simulink model "sl_fforward"  (Simulink 7.6)
settings: Solver=ode45  StartTime=0.0  StopTime=10.0  RelTol=1e-3
undefined symbols (not defined in the file or in its folder): p560
libraries: roblocks x4
settings Model: Creator=corkep  LastModifiedBy=n6334687

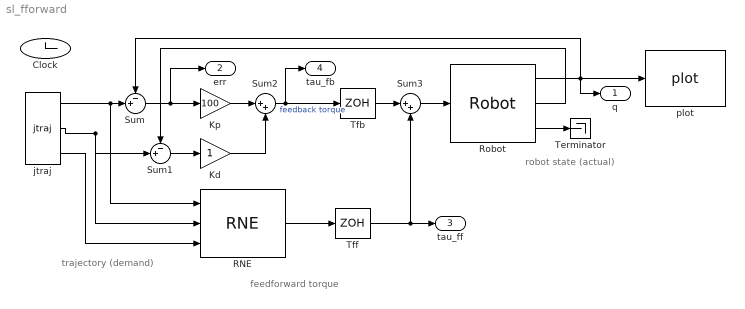
== system sl_fforward ==
  note: trajectory
      | (demand)
  note: robot state
      | (actual)
  note: feedforward torque
  Clock : Clock
      settings: Decimation=10
  Kd : Gain  SaturateOnIntegerOverflow=on  OutDataTypeStr=Inherit: Same as input  ParamDataTypeStr=Inherit: Same as input
  Kp : Gain  Gain=100  SaturateOnIntegerOverflow=on  OutDataTypeStr=Inherit: Same as input  ParamDataTypeStr=Inherit: Same as input
  RNE : roblocks/Dynamics/RNE  SystemSampleTime=-1  robot=p560.nofriction()  grav=[0 0 9.81]
  Robot : roblocks/Dynamics/Robot  SystemSampleTime=-1  robot=p560  q0=[0 0 0 0 0 0]
  Sum : Sum  Inputs=-+|  SaturateOnIntegerOverflow=on  InputSameDT=on  OutDataTypeStr=Inherit: Same as first input
  Sum1 : Sum  Inputs=-+|  SaturateOnIntegerOverflow=on  InputSameDT=on  OutDataTypeStr=Inherit: Same as first input
  Sum2 : Sum  Inputs=|++  SaturateOnIntegerOverflow=on  InputSameDT=on  OutDataTypeStr=Inherit: Same as first input
  Sum3 : Sum  Inputs=|++  SaturateOnIntegerOverflow=on  InputSameDT=on  OutDataTypeStr=Inherit: Same as first input
  Terminator : Terminator
  Tfb : ZeroOrderHold  SampleTime=0.01
  Tff : ZeroOrderHold  SampleTime=0.01
  jtraj : roblocks/Trajectory/jtraj  SystemSampleTime=-1  q0=[0 0 0 0 0 0]  qf=[pi/4 pi/2 -pi/2 0 0 0]  tmax=10
  plot : roblocks/Robot Graphics/plot  SystemSampleTime=-1  robot=p560
  q : Outport
  err : Outport  Port=2
  tau_ff : Outport  Port=3
  tau_fb : Outport  Port=4
  wires:
  Kd/1 -> Sum2/2
  Sum/1 -> Kp/1, err/1
  Kp/1 -> Sum2/1
  Sum1/1 -> Kd/1
  Sum2/1 -> Tfb/1, tau_fb/1  "feedback torque"
  Sum3/1 -> Robot/1
  Robot/1 -> plot/1, Sum/1, q/1
  Robot/2 -> Sum1/1
  jtraj/1 -> Sum/2, RNE/1
  jtraj/2 -> Sum1/2, RNE/2
  jtraj/3 -> RNE/3
  Robot/3 -> Terminator/1
  Tff/1 -> Sum3/2, tau_ff/1
  Tfb/1 -> Sum3/1
  RNE/1 -> Tff/1
